simulink model "TestPFCStage"  (R2025b)
settings: Solver=ode23t  StartTime=0.0  StopTime=3.0  MaxStep=1e-4  RelTol=1e-4
libraries: fl_lib x12, nesl_utility x6, datacenter_lib x1
settings Model: Creator=saprasad  LastModifiedBy=saprasad
settings SimscapeCC: SimscapeLogType=all  SimscapeLogName=simlog_TestPFCStage  SimscapeLogLimitData=off

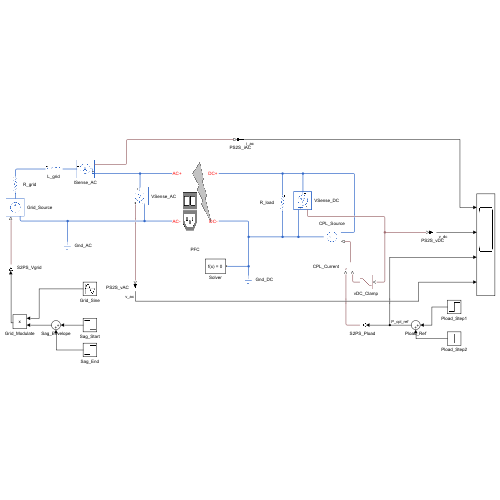
[thumbnail: Simulink's stored preview of the top-level diagram]
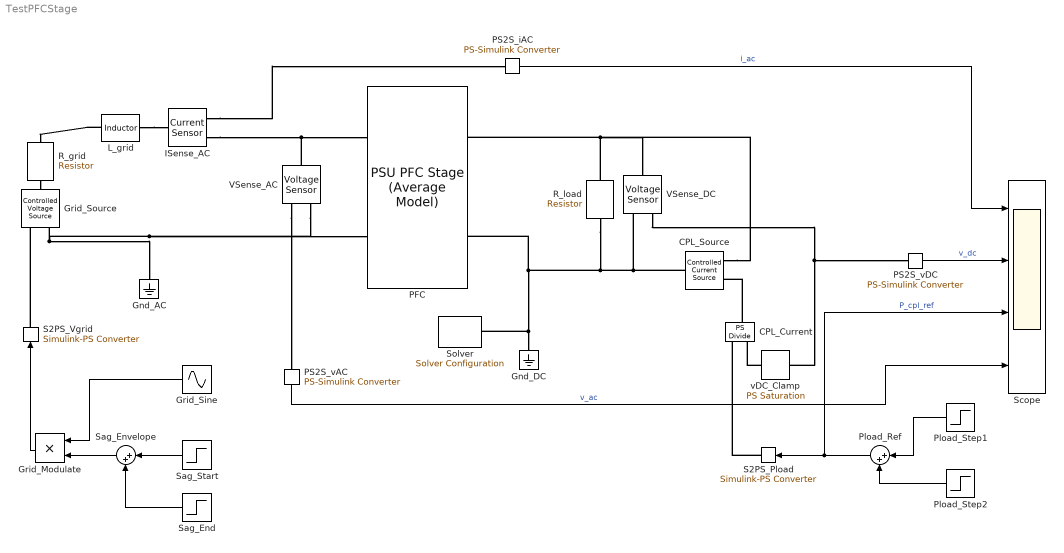
== system TestPFCStage ==
  CPL_Current : fl_lib/Physical Signals/Functions/PS Divide
  CPL_Source : fl_lib/Electrical/Electrical Sources/Controlled Current Source
  Gnd_AC : fl_lib/Electrical/Electrical Elements/Electrical Reference
  Gnd_DC : fl_lib/Electrical/Electrical Elements/Electrical Reference
  Grid_Modulate : Product
  Grid_Sine : Sin  Amplitude=678.8225099390857  Frequency=376.99111843077515  SampleTime=0
  Grid_Source : fl_lib/Electrical/Electrical Sources/Controlled Voltage Source
  ISense_AC : fl_lib/Electrical/Electrical Sensors/Current Sensor
  L_grid : fl_lib/Electrical/Electrical Elements/Inductor  l=5e-5 H  r=1e-6 Ohm  g=1e-9 1/Ohm  i_specify=off  i_priority=None  i=0 A  i_nominal_specify=off  i_nominal_value=1  i_nominal_unit=A  v_specify=off  v_priority=None  v=0 V  v_nominal_specify=off  v_nominal_value=1  v_nominal_unit=V  i_L_specify=off  i_L_priority=High  i_L=0 A  i_L_nominal_specify=off  i_L_nominal_value=1  i_L_nominal_unit=A
  PFC : datacenter_lib/PSU PFC Stage (Average Model)  C_dc=0.03 F  V_dc_ref=400 V  Kp_pfc=200 W/V  Ki_pfc=600 W/(V*s)  eta_pfc=0.97  P_max=20000 W  G_damp=0.002 1/Ohm  tau_rms=0.04 s  V_nom=480 V  L_ac=0.5e-3 H  R_ac=0.01 Ohm  i_ac_specify=off  i_ac_priority=None  i_ac=0 A  i_ac_nominal_specify=off  i_ac_nominal_value=1  i_ac_nominal_unit=A  v_ac_specify=off  v_ac_priority=Low  v_ac=480 V  v_ac_nominal_specify=off  v_ac_nominal_value=1  v_ac_nominal_unit=V  v_dc_specify=on  v_dc_priority=High  v_dc=400 V  v_dc_nominal_specify=off  v_dc_nominal_value=1  v_dc_nominal_unit=V  i_dc_specify=off  i_dc_priority=None  i_dc=0 A  i_dc_nominal_specify=off  i_dc_nominal_value=1  i_dc_nominal_unit=A  pfc_integrator_specify=on  pfc_integrator_priority=Low  pfc_integrator=0 V*s  pfc_integrator_nominal_specify=off  pfc_integrator_nominal_value=1  pfc_integrator_nominal_unit=V*s  v_rms_sq_specify=off  v_rms_sq_priority=Low  v_rms_sq=230400 V^2  v_rms_sq_nominal_specify=off  v_rms_sq_nominal_value=1  v_rms_sq_nominal_unit=V^2
      settings: InternalSimscapePortConfiguration="{\"Bottom\":[],\"Left\":[{\"id\":\"p\",\"label\":\"AC+\",\"type\":\"foundation.electrical.electrical\"},{\"id\":\"n\",\"label\":\"AC-\",\"type\":\"foundation.electrical.electrical\"}],\"Right\":[{\"id\":\"dc_p\",\"label\":\"DC+\",\"type\":\"foundation.electrical.electrical\"},{\"id\":\"dc_n\",\"label\":\"DC-\",\"type\":\"foundation.electrical.electrical\"}],\"Top\":[]}"
  PS2S_iAC : nesl_utility/PS-Simulink Converter  PhysicalDomain=network_engine_domain  SubClassName=ps_output  LeftPortType=input  RightPortType=output  PseudoPeriodic=off  Frequencies=[]  VectorFormat=inherit  Unit=A  AffineConversion=off
  PS2S_vAC : nesl_utility/PS-Simulink Converter  PhysicalDomain=network_engine_domain  SubClassName=ps_output  LeftPortType=input  RightPortType=output  PseudoPeriodic=off  Frequencies=[]  VectorFormat=inherit  Unit=V  AffineConversion=off
  PS2S_vDC : nesl_utility/PS-Simulink Converter  PhysicalDomain=network_engine_domain  SubClassName=ps_output  LeftPortType=input  RightPortType=output  PseudoPeriodic=off  Frequencies=[]  VectorFormat=inherit  Unit=V  AffineConversion=off
  Pload_Ref : Sum  Inputs=|++
  Pload_Step1 : Step  Time=1.0  Before=4000  After=8000  SampleTime=0
  Pload_Step2 : Step  Time=1.5  After=4000  SampleTime=0
  R_grid : fl_lib/Electrical/Electrical Elements/Resistor  R=0.02 Ohm  i_specify=off  i_priority=None  i=0 A  i_nominal_specify=off  i_nominal_value=1  i_nominal_unit=A  v_specify=off  v_priority=None  v=0 V  v_nominal_specify=off  v_nominal_value=1  v_nominal_unit=V
  R_load : fl_lib/Electrical/Electrical Elements/Resistor  R=40 Ohm  i_specify=off  i_priority=None  i=0 A  i_nominal_specify=off  i_nominal_value=1  i_nominal_unit=A  v_specify=off  v_priority=None  v=0 V  v_nominal_specify=off  v_nominal_value=1  v_nominal_unit=V
  S2PS_Pload : nesl_utility/Simulink-PS Converter  PhysicalDomain=network_engine_domain  SubClassName=ps_input  LeftPortType=input  RightPortType=output  PseudoPeriodic=off  Frequencies=[]  NoiseDistribution=none  NoiseParameters=[]  Unit=W  AffineConversion=off  FilteringAndDerivatives=provide  SimscapeFilterOrder=1  InputFilterTimeConstant=0.001  UdotUserProvided=0
  S2PS_Vgrid : nesl_utility/Simulink-PS Converter  PhysicalDomain=network_engine_domain  SubClassName=ps_input  LeftPortType=input  RightPortType=output  PseudoPeriodic=off  Frequencies=[]  NoiseDistribution=none  NoiseParameters=[]  Unit=V  AffineConversion=off  FilteringAndDerivatives=provide  SimscapeFilterOrder=1  InputFilterTimeConstant=0.001  UdotUserProvided=0
  Sag_End : Step  Time=2.3  After=0.4  SampleTime=0
  Sag_Envelope : Sum  Inputs=|++
  Sag_Start : Step  Time=2.0  Before=1  After=0.6  SampleTime=0
  Scope : Scope  NumInputPorts=4
      settings: ActiveDisplayYMinimum=-121.37737135826985  ActiveDisplayYMaximum=146.67494485924317
  Solver : nesl_utility/Solver Configuration  PhysicalDomain=network_engine_domain  SubClassName=solver  LeftPortType=input  RightPortType=generic  Tones=[]  Harmonics=[]  SimulateNoise=off  Profile=off  UseLocalSampling=off  EnableSwitchedLinearOptims=on  FrequencyDomain=off  UseCCode=off  RelTol=0.001  AbsTol=0.001  MinStep=1e-09  ToWorkspace=off  RevertToSquareIcSolve=off  NumHomotopyIterations=100  PhasorMode=off  PhasorModeNumHarmonics=1  ConsistencySolver=NEWTON_XTOL_AFTER_FTOL  IndexReductionMethod=DerivativeReplacement  DoDC=off  ResidualTolerance=1e-7  ConsistencyTolSource=GLOBAL  ConsistencyAbsTol=0.001  ConsistencyRelTol=0.001  ConsistencyTolFactor=1e3  UseLocalSolver=off  LocalSolverChoice=NE_BACKWARD_EULER_ADVANCER  ResolveIndetEquations=on  FunctionEvalNumThread=1  LocalSolverSampleTime=5e-5  DoFixedCost=off  MaxNonlinIter=3  MaxModeIter=2  ComputeImpulses=off  ImpulseIterations=2  LinearAlgebra=auto  LinearAlgebraNumThread=0  EquationFormulation=NE_TIME_EF  DelaysMemoryBudget=1024  AutomaticFiltering=on  FilteringTimeConstant=0.001  PartitionStorageMethod=AS_NEEDED  PartitionMemoryBudget=1024  PartitionMethod=ROBUST  MultibodyUseLocalSolver=off  MultibodyLocalSolverChoice=ODE1  MultibodyLocalSolverSampleTime=0.001
  VSense_AC : fl_lib/Electrical/Electrical Sensors/Voltage Sensor
  VSense_DC : fl_lib/Electrical/Electrical Sensors/Voltage Sensor
  vDC_Clamp : fl_lib/Physical Signals/Nonlinear Operators/PS Saturation  upper_limit=800 V  lower_limit=200 V  ZeroCross=false
  wires:
  Sag_Start/1 -> Sag_Envelope/1
  Sag_End/1 -> Sag_Envelope/2
  Grid_Sine/1 -> Grid_Modulate/1
  Sag_Envelope/1 -> Grid_Modulate/2
  Grid_Modulate/1 -> S2PS_Vgrid/1
  Pload_Step1/1 -> Pload_Ref/1
  Pload_Step2/1 -> Pload_Ref/2
  Pload_Ref/1 -> Scope/3, S2PS_Pload/1  "P_cpl_ref"
  PS2S_iAC/1 -> Scope/1  "i_ac"
  PS2S_vDC/1 -> Scope/2  "v_dc"
  PS2S_vAC/1 -> Scope/4  "v_ac"
  connections:
  ISense_AC/RConn2 -- VSense_AC/LConn1 -- PFC/LConn1
  Grid_Source/RConn2 -- VSense_AC/RConn2 -- PFC/LConn2 -- Gnd_AC/LConn1
  CPL_Source/LConn1 -- R_load/RConn1 -- Gnd_DC/LConn1 -- Solver/RConn1 -- PFC/RConn2 -- VSense_DC/RConn2
  L_grid/LConn1 -- R_grid/RConn1
  L_grid/RConn1 -- ISense_AC/LConn1
  R_load/LConn1 -- CPL_Source/RConn2 -- VSense_DC/LConn1 -- PFC/RConn1
  S2PS_Vgrid/RConn1 -- Grid_Source/RConn1
  S2PS_Pload/RConn1 -- CPL_Current/LConn1
  CPL_Current/RConn1 -- CPL_Source/RConn1
  VSense_AC/RConn1 -- PS2S_vAC/LConn1
  ISense_AC/RConn1 -- PS2S_iAC/LConn1
  R_grid/LConn1 -- Grid_Source/LConn1
  VSense_DC/RConn1 -- PS2S_vDC/LConn1 -- vDC_Clamp/LConn1
  vDC_Clamp/RConn1 -- CPL_Current/LConn2
